simulink model "C2_Wideband_Filter"  (R2019b)
settings: Solver=VariableStepAuto  StartTime=0.0  StopTime=testtime  RelTol=1e-3
InitFcn:
  | C2_Wideband_Test_Parameters
StopFcn:
  | Verify_C2_Wideband_Filter
values from neighbouring files (symbols this model uses):
  Fs = 48e3    (= 48000)    [C2_Wideband_Test_Parameters.m]
undefined symbols (not defined in the file or in its folder): C2coeffs, dfilt, norm_gainc2
libraries: dsparch4 x2, dspsrcs4 x2
settings Model: Creator=mblun  LastModifiedBy=t96f346
settings OptimizationCC: BlockReduction=off  ConditionallyExecuteInputs=off  DefaultParameterBehavior=Inlined
settings DebuggingCC: AlgebraicLoopMsg=error
settings HardwareCC: ProdBitPerPointer=32  ProdBitPerSizeT=32  ProdBitPerPtrDiffT=32  ProdLargestAtomicFloat=None  ProdIntDivRoundTo=Undefined  ProdEndianess=Unspecified  ProdWordSize=32  ProdHWDeviceType=ASIC/FPGA->ASIC/FPGA  TargetBitPerPointer=64  TargetBitPerSizeT=64  TargetBitPerPtrDiffT=64  TargetLongLongMode=on  TargetIntDivRoundTo=Zero  TargetEndianess=LittleEndian  TargetWordSize=64  TargetHWDeviceType=Custom Processor->MATLAB Host Computer  ProdEqTarget=off
settings SFSimCC: CustomCodeUndefinedFunction=UseInterfaceOnly

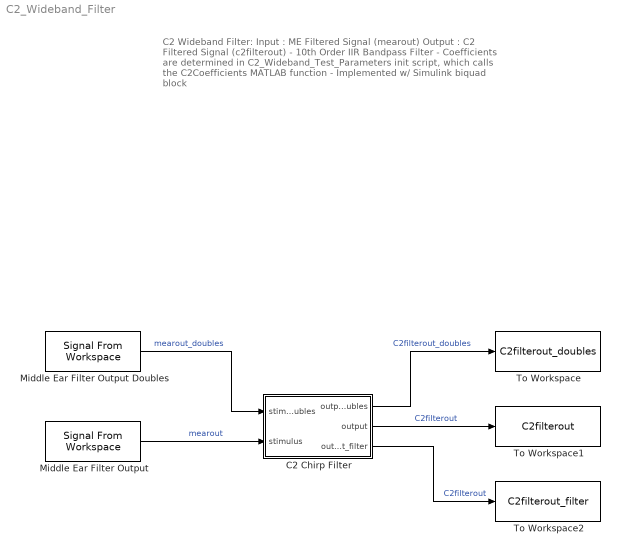
== system C2_Wideband_Filter ==
  note: C2 Wideband Filter:
      |
      | Input : ME Filtered Signal (mearout)
      |
      | Output : C2 Filtered Signal (c2filterout)
      |
      | - 10th Order IIR Bandpass Filter
      |
      | - Coefficients are determined in C2_Wideband_Test_Parameters init script, which calls the C2Coefficients MATLAB function
      |
      | - Implemented w/ Simulink biquad block
  C2 Chirp Filter : Subsystem
  Middle Ear Filter Output : dspsrcs4/Signal From Workspace  X=RxSignal  Ts=1/Fs  nsamps=1  OutputAfterFinalValue=Setting to zero  ignoreOrWarnInputAndFrameLengths=off  OutputFrames=off
  Middle Ear Filter Output Doubles : dspsrcs4/Signal From Workspace  X=RxSignal_doubles  Ts=1/Fs  nsamps=1  OutputAfterFinalValue=Setting to zero  ignoreOrWarnInputAndFrameLengths=off  OutputFrames=off
  To Workspace : ToWorkspace  VariableName=C2filterout_doubles  SampleTime=-1
      settings: Save2DSignal=2-D array (concatenate along first dimension)
  To Workspace1 : ToWorkspace  VariableName=C2filterout  SampleTime=-1
      settings: Save2DSignal=2-D array (concatenate along first dimension)
  To Workspace2 : ToWorkspace  VariableName=C2filterout_filter  SampleTime=-1
      settings: Save2DSignal=2-D array (concatenate along first dimension)
  wires:
  Middle Ear Filter Output Doubles/1 -> C2 Chirp Filter/1(stimulus_doubles)  "mearout_doubles"
  C2 Chirp Filter/2(output) -> To Workspace1/1  "C2filterout"
  Middle Ear Filter Output/1 -> C2 Chirp Filter/2(stimulus)  "mearout"
  C2 Chirp Filter/1(output_doubles) -> To Workspace/1  "C2filterout_doubles"
  C2 Chirp Filter/3(output_filter) -> To Workspace2/1  "C2filterout"

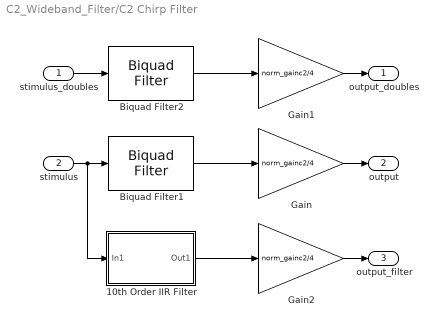
== system C2_Wideband_Filter/C2 Chirp Filter ==
  stimulus_doubles : Inport
  stimulus : Inport  Port=2
  10th Order IIR Filter : Subsystem
  Biquad Filter1 : dsparch4/Biquad Filter  FilterSource=Dialog parameters  CoeffSource=Specify via dialog  FilterObject=dfilt.df2tsos([1 0.3 0.4],[1 0.1 0.2])  IIRFiltStruct=Direct form I  BiQuadCoeffs=C2coeffs  ScaleValues=1  IC=0  ICnum=0  ICden=0  a0Flag=Warning  optimizeScaleValues=on  ScaleValueMode=Specify via input port (g)  roundingMode=Floor  overflowMode=on  scaleValueFracLength=14  denProdOutputFracLength=30  denAccumFracLength=30  secondMemoryFracLength=15
      settings: SourceProductName=DSP System Toolbox
  Biquad Filter2 : dsparch4/Biquad Filter  FilterSource=Dialog parameters  CoeffSource=Specify via dialog  FilterObject=dfilt.df2tsos([1 0.3 0.4],[1 0.1 0.2])  IIRFiltStruct=Direct form I  BiQuadCoeffs=C2coeffs  ScaleValues=1  IC=0  ICnum=0  ICden=0  a0Flag=Warning  optimizeScaleValues=on  ScaleValueMode=Specify via input port (g)  roundingMode=Floor  overflowMode=on  scaleValueFracLength=14  denProdOutputFracLength=30  denAccumFracLength=30  secondMemoryFracLength=15
      settings: SourceProductName=DSP System Toolbox
  Gain : Gain  Gain=norm_gainc2/4
  Gain1 : Gain  Gain=norm_gainc2/4
  Gain2 : Gain  Gain=norm_gainc2/4
  output_doubles : Outport  VectorParamsAs1DForOutWhenUnconnected=off
  output : Outport  Port=2  VectorParamsAs1DForOutWhenUnconnected=off
  output_filter : Outport  Port=3  VectorParamsAs1DForOutWhenUnconnected=off
  wires:
  stimulus/1 -> 10th Order IIR Filter/1(In1), Biquad Filter1/1
  Biquad Filter1/1 -> Gain/1
  Gain/1 -> output/1
  stimulus_doubles/1 -> Biquad Filter2/1
  Gain1/1 -> output_doubles/1
  Biquad Filter2/1 -> Gain1/1
  10th Order IIR Filter/1(Out1) -> Gain2/1
  Gain2/1 -> output_filter/1

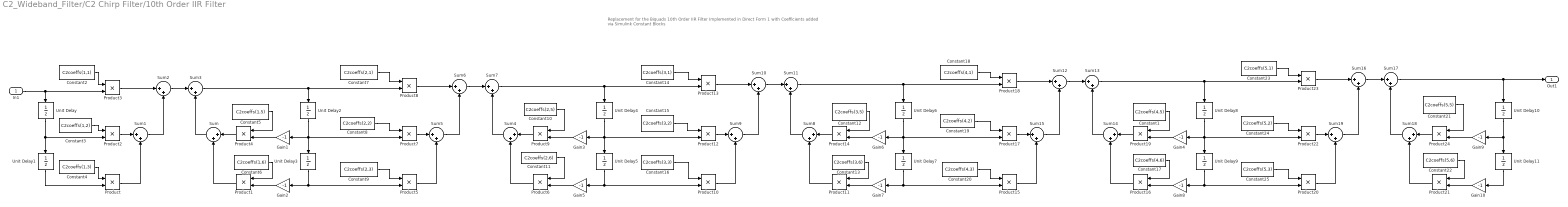
== system C2_Wideband_Filter/C2 Chirp Filter/10th Order IIR Filter ==
  note: Replacement for the Biquads
      | 10th Order IIR Filter Implemented in Direct Form 1 with Coefficients added via Simulink Constant Blocks
  In1 : Inport  OutDataTypeStr=single
  Constant1 : Constant  Value=C2coeffs(4,5)  OutDataTypeStr=single  SampleTime=-1
  Constant10 : Constant  Value=C2coeffs(2,5)  OutDataTypeStr=single  SampleTime=-1
  Constant11 : Constant  Value=C2coeffs(2,6)  OutDataTypeStr=single  SampleTime=-1
  Constant12 : Constant  Value=C2coeffs(3,5)  OutDataTypeStr=single  SampleTime=-1
  Constant13 : Constant  Value=C2coeffs(3,6)  OutDataTypeStr=single  SampleTime=-1
  Constant14 : Constant  Value=C2coeffs(3,1)  OutDataTypeStr=single  SampleTime=-1
  Constant15 : Constant  Value=C2coeffs(3,2)  OutDataTypeStr=single  SampleTime=-1
  Constant16 : Constant  Value=C2coeffs(3,3)  OutDataTypeStr=single  SampleTime=-1
  Constant17 : Constant  Value=C2coeffs(4,6)  OutDataTypeStr=single  SampleTime=-1
  Constant18 : Constant  Value=C2coeffs(4,1)  OutDataTypeStr=single  SampleTime=-1
  Constant19 : Constant  Value=C2coeffs(4,2)  OutDataTypeStr=single  SampleTime=-1
  Constant2 : Constant  Value=C2coeffs(1,1)  OutDataTypeStr=single  SampleTime=-1
  Constant20 : Constant  Value=C2coeffs(4,3)  OutDataTypeStr=single  SampleTime=-1
  Constant21 : Constant  Value=C2coeffs(5,5)  OutDataTypeStr=single  SampleTime=-1
  Constant22 : Constant  Value=C2coeffs(5,6)  OutDataTypeStr=single  SampleTime=-1
  Constant23 : Constant  Value=C2coeffs(5,1)  OutDataTypeStr=single  SampleTime=-1
  Constant24 : Constant  Value=C2coeffs(5,2)  OutDataTypeStr=single  SampleTime=-1
  Constant25 : Constant  Value=C2coeffs(5,3)  OutDataTypeStr=single  SampleTime=-1
  Constant3 : Constant  Value=C2coeffs(1,2)  OutDataTypeStr=single  SampleTime=-1
  Constant4 : Constant  Value=C2coeffs(1,3)  OutDataTypeStr=single  SampleTime=-1
  Constant5 : Constant  Value=C2coeffs(1,5)  OutDataTypeStr=single  SampleTime=-1
  Constant6 : Constant  Value=C2coeffs(1,6)  OutDataTypeStr=single  SampleTime=-1
  Constant7 : Constant  Value=C2coeffs(2,1)  OutDataTypeStr=single  SampleTime=-1
  Constant8 : Constant  Value=C2coeffs(2,2)  OutDataTypeStr=single  SampleTime=-1
  Constant9 : Constant  Value=C2coeffs(2,3)  OutDataTypeStr=single  SampleTime=-1
  Gain{1..10} (10 alike) : Gain  Gain=-1
  Product{,1..24} (25 alike) : Product
  Sum{,1..19} (20 alike) : Sum  Inputs=|++
  Unit Delay{,1..11} (12 alike) : UnitDelay  SampleTime=-1  HasFrameUpgradeWarning=on
  Out1 : Outport  OutDataTypeStr=single
  wires:
  Sum5/1 -> Sum6/2
  Product/1 -> Sum1/2
  Constant6/1 -> Product1/1
  Sum1/1 -> Sum2/2
  Sum6/1 -> Sum7/1
  Sum2/1 -> Sum3/1
  Constant8/1 -> Product7/1
  Sum14/1 -> Sum13/2
  Constant10/1 -> Product9/1
  Product5/1 -> Sum5/2
  Product2/1 -> Sum1/1
  Gain10/1 -> Product21/2
  Constant5/1 -> Product4/1
  Unit Delay11/1 -> Gain10/1
  Constant4/1 -> Product/1
  Sum4/1 -> Sum7/2
  Constant18/1 -> Product18/1
  Constant12/1 -> Product14/1
  Product4/1 -> Sum/1
  Product17/1 -> Sum15/1
  Constant14/1 -> Product13/1
  Gain2/1 -> Product1/2
  Sum17/1 -> Unit Delay10/1, Out1/1
  Product13/1 -> Sum10/1
  Sum15/1 -> Sum12/2
  Product10/1 -> Sum9/2
  Gain3/1 -> Product9/2
  Unit Delay/1 -> Unit Delay1/1, Product2/2
  Unit Delay8/1 -> Product22/2, Unit Delay9/1, Gain4/1
  Sum19/1 -> Sum16/2
  Constant16/1 -> Product10/1
  Product9/1 -> Sum4/1
  Sum3/1 -> Unit Delay2/1, Product8/2
  Product23/1 -> Sum16/1
  Product3/1 -> Sum2/1
  Product20/1 -> Sum19/2
  Constant3/1 -> Product2/1
  Constant21/1 -> Product24/1
  Unit Delay2/1 -> Product7/2, Unit Delay3/1, Gain1/1
  Unit Delay7/1 -> Product15/2, Gain7/1
  Constant19/1 -> Product17/1
  Constant9/1 -> Product5/1
  Sum16/1 -> Sum17/1
  Constant22/1 -> Product21/1
  Constant15/1 -> Product12/1
  Product18/1 -> Sum12/1
  Constant13/1 -> Product11/1
  Sum11/1 -> Unit Delay6/1, Product18/2
  Sum/1 -> Sum3/2
  Unit Delay6/1 -> Product17/2, Unit Delay7/1, Gain6/1
  Unit Delay10/1 -> Unit Delay11/1, Gain9/1
  Gain9/1 -> Product24/2
  Gain5/1 -> Product6/2
  Product14/1 -> Sum8/1
  Sum10/1 -> Sum11/1
  Gain4/1 -> Product19/2
  Sum8/1 -> Sum11/2
  Constant17/1 -> Product16/1
  Gain1/1 -> Product4/2
  Sum9/1 -> Sum10/2
  Gain7/1 -> Product11/2
  Product6/1 -> Sum4/2
  Unit Delay1/1 -> Product/2
  Sum7/1 -> Unit Delay4/1, Product13/2
  Constant11/1 -> Product6/1
  Constant25/1 -> Product20/1
  Sum13/1 -> Unit Delay8/1, Product23/2
  Unit Delay5/1 -> Product10/2, Gain5/1
  Product16/1 -> Sum14/2
  Gain6/1 -> Product14/2
  Product7/1 -> Sum5/1
  Product22/1 -> Sum19/1
  Product15/1 -> Sum15/2
  Unit Delay3/1 -> Product5/2, Gain2/1
  Product11/1 -> Sum8/2
  Constant24/1 -> Product22/1
  Sum18/1 -> Sum17/2
  Constant20/1 -> Product15/1
  Product12/1 -> Sum9/1
  Unit Delay9/1 -> Product20/2, Gain8/1
  Unit Delay4/1 -> Product12/2, Unit Delay5/1, Gain3/1
  Constant1/1 -> Product19/1
  Product8/1 -> Sum6/1
  Gain8/1 -> Product16/2
  In1/1 -> Product3/2, Unit Delay/1
  Constant7/1 -> Product8/1
  Constant2/1 -> Product3/1
  Product21/1 -> Sum18/2
  Constant23/1 -> Product23/1
  Product24/1 -> Sum18/1
  Product1/1 -> Sum/2
  Product19/1 -> Sum14/1
  Sum12/1 -> Sum13/1
